simulink model "Overall"  (R2020a)
settings: Solver=VariableStepAuto  StartTime=0.0  StopTime=240  RelTol=1e-3
settings Model: Creator=Ricky  LastModifiedBy=noel

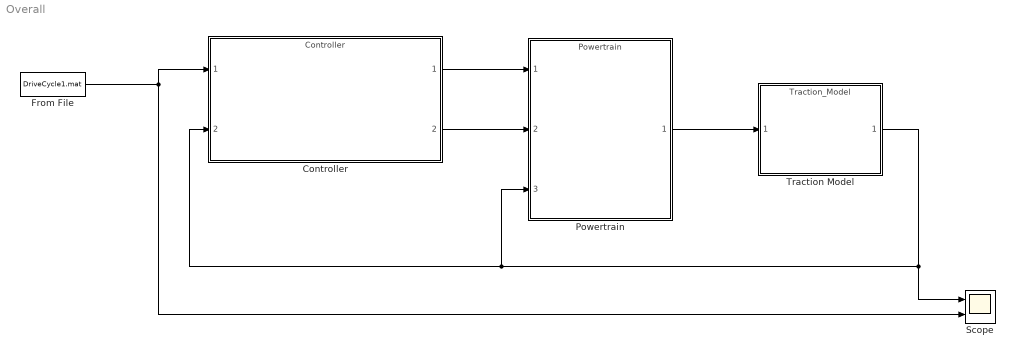
== system Overall ==
  Controller : ModelReference  ModelNameDialog=Controller.slx  SimulationMode=Normal  ModelReferenceVersion=1.2
  From File : FromFile  FileName=DriveCycle1.mat  SampleTime=0
  Powertrain : ModelReference  ModelNameDialog=Powertrain.slx  SimulationMode=Normal  ModelReferenceVersion=1.3
  Scope : Scope  NumInputPorts=2
  Traction Model : ModelReference  ModelNameDialog=Traction_Model.slx  SimulationMode=Normal  ModelReferenceVersion=1.17
  wires:
  Traction Model/1 -> Powertrain/3, Controller/2, Scope/1
  From File/1 -> Controller/1, Scope/2
  Controller/1 -> Powertrain/1
  Controller/2 -> Powertrain/2
  Powertrain/1 -> Traction Model/1
